simulink model "ControllerModelStateflow"  (R2022b)
settings: Solver=VariableStepAuto  StartTime=0.0  StopTime=inf  RelTol=1e-3
libraries: slpidlib x1
settings Model: Creator=steph  LastModifiedBy=steph
settings OptimizationCC: BlockReduction=off  DefaultParameterBehavior=Inlined  BufferReuse=off

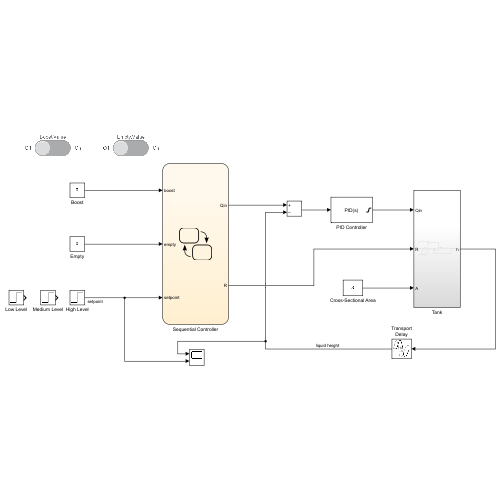
[thumbnail: Simulink's stored preview of the top-level diagram]
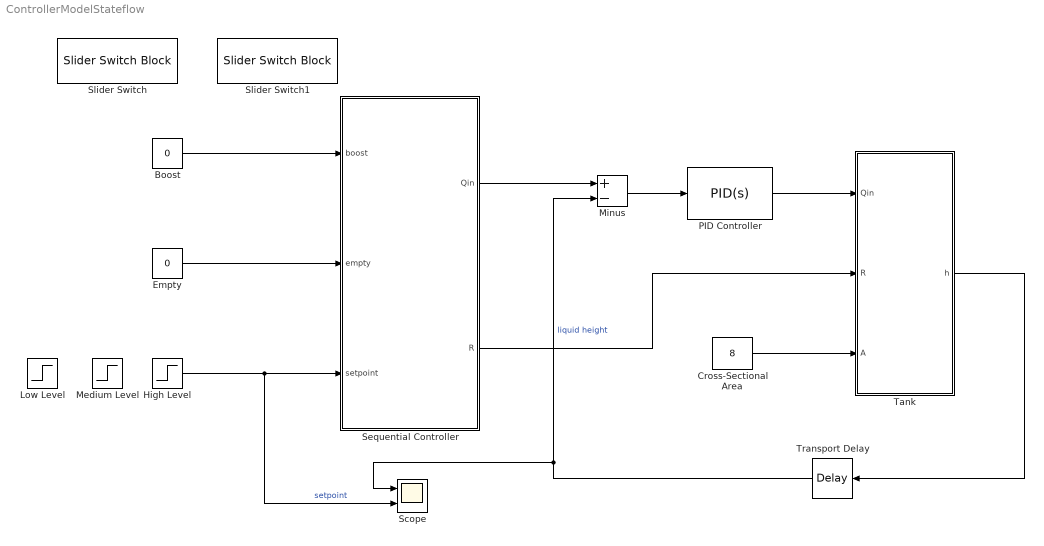
== system ControllerModelStateflow ==
  Boost : Constant  Value=0  OutMin=0  OutMax=1
  Cross-Sectional Area : Constant  Value=8  OutMin=0  OutMax=200
  Empty : Constant  Value=0  OutMin=0  OutMax=1
  High Level : Step  Time=4  After=16  SampleTime=0
  Low Level : Step  Time=0.25  After=2  SampleTime=0
  Medium Level : Step  Time=2  After=8  SampleTime=0
  Minus : Sum  Inputs=+-
  PID Controller : slpidlib/PID Controller  Controller=PID  Form=Parallel  TimeDomain=Continuous-time  UseExternalTs=off  SampleTime=-1  IntegratorMethod=Forward Euler  FilterMethod=Forward Euler  ControllerParametersSource=internal  P=0.6*8.25  I=2*(1/6.5)  UseKiTs=off  D=0.125/(1/2.3)  N=100  UseFilter=on  TunerSelectOption=Transfer Function Based (PID Tuner App)  InitialConditionSource=internal  InitialConditionForIntegrator=0  InitialConditionForFilter=0  DifferentiatorICPrevScaledInput=0  ExternalReset=none  TrackingMode=off  Kt=1  LimitOutput=on  SatLimitsSource=internal  UpperSaturationLimit=50  LowerSaturationLimit=0  LinearizeAsGain=on  AntiWindupMode=none  Kb=1  LimitIntegrator=off  UpperIntegratorSaturationLimit=inf  LowerIntegratorSaturationLimit=-inf  POutMin=[]  POutMax=[]  IOutMin=[]  IOutMax=[]  DOutMin=[]  DOutMax=[]  NOutMin=[]  NOutMax=[]  SumOutMin=[]  SumOutMax=[]  SaturationOutMin=[]  SaturationOutMax=[]  PParamMin=[]  PParamMax=[]  IParamMin=[]  IParamMax=[]  DParamMin=[]  DParamMax=[]  NParamMin=[]  NParamMax=[]  KbParamMin=[]  KbParamMax=[]  KtParamMin=[]  KtParamMax=[]  KbOutMin=[]  KbOutMax=[]  KtOutMin=[]  KtOutMax=[]  IntegratorOutMin=[]  IntegratorOutMax=[]  FilterOutMin=[]  FilterOutMax=[]  SumI1OutMin=[]  SumI1OutMax=[]  SumI2OutMin=[]  SumI2OutMax=[]  SumI3OutMin=[]  SumI3OutMax=[]  SumI4OutMin=[]  SumI4OutMax=[]  SumDOutMin=[]  SumDOutMax=[]  DifferentiatorOutMin=[]  DifferentiatorOutMax=[]  FilterDiffOutCoefMin=[]  FilterDiffOutCoefMax=[]  ReciprocalOutMin=[]  ReciprocalOutMax=[]  SumDenOutMin=[]  SumDenOutMax=[]  SumNumOutMin=[]  SumNumOutMax=[]  DivideOutMin=[]  DivideOutMax=[]  UdiffTsProdOutMin=[]  UdiffTsProdOutMax=[]  NTsProdOutMin=[]  NTsProdOutMax=[]  UintegralTsProdOutMin=[]  UintegralTsProdOutMax=[]  UngainTsProdOutMin=[]  UngainTsProdOutMax=[]  ClampingZeroOutDataTypeStr=Inherit: Inherit via back propagation  ClampingZeroOutMin=[]  ClampingZeroOutMax=[]  FilterDenConstantOutDataTypeStr=Inherit: Inherit via back propagation  FilterDenConstantOutMin=[]  FilterDenConstantOutMax=[]  PCopyOutDataTypeStr=Inherit: Inherit via back propagation  PCopyOutMin=[]  PCopyOutMax=[]  NCopyOutDataTypeStr=Inherit: Inherit via back propagation  NCopyOutMin=[]  NCopyOutMax=[]  IntegratorContinuousStateAttributes=''  IntegratorStateMustResolveToSignalObject=off  IntegratorRTWStateStorageClass=Auto  FilterContinuousStateAttributes=''  FilterStateMustResolveToSignalObject=off  FilterRTWStateStorageClass=Auto  ParallelPVariant=InternalParameters  IdealPVariant=Disabled  IVariant=InternalParameters  DVariant=InternalParameters  IntegratorVariant=Continuous  SatVariant=Enabled  AWVariant=Passthrough  PCopyVariant=Disabled  TRVariant=Disabled  FdbkBlocksVariant=Forward  IdealPFdbkVariant=Disabled  SatFdbkVariant=Disabled  DerivativeFilterVariant=ContFilter  NVariant=InternalParameters  NCopyVariant=Disabled  FilterICVariant=InternalICsFilter  IntegratorICVariant=InternalICs  ExternalResetVariant=Disabled  TRSumVariant=Passthrough  SumFdbkVariant=Disabled  SumVariant=Sum_PID  TsampFilterVariant=InternalTs  TsampNgainVariant=Passthrough  TsampIntegralVariant=Passthrough  ExternalSaturationOutDataTypeStr=Inherit: Same as second input
  Scope : Scope  NumInputPorts=2
  Sequential Controller : Stateflow chart  TreatAsAtomicUnit=on
  Slider Switch : SliderSwitchBlock
      settings: Values={{'Off', 'On'}, [0 1]}
  Slider Switch1 : SliderSwitchBlock
      settings: Values={{'Off', 'On'}, [0 1]}
  Tank : Subsystem
  Transport Delay : TransportDelay  DelayTime=0.05
  wires:
  Sequential Controller/2(R) -> Tank/2(R)
  Cross-Sectional Area/1 -> Tank/3(A)
  Tank/1(h) -> Transport Delay/1
  Transport Delay/1 -> Minus/2, Scope/1  "liquid height"
  Minus/1 -> PID Controller/1
  PID Controller/1 -> Tank/1(Qin)
  Sequential Controller/1(Qin) -> Minus/1
  Boost/1 -> Sequential Controller/1(boost)
  Empty/1 -> Sequential Controller/2(empty)
  High Level/1 -> Scope/2, Sequential Controller/3(setpoint)  "setpoint"

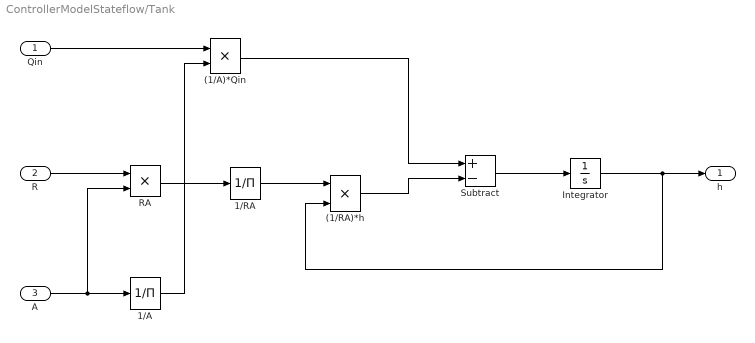
== system ControllerModelStateflow/Tank ==
  Qin : Inport
  R : Inport  Port=2
  A : Inport  Port=3
  (1/A)*Qin : Product
  (1/RA)*h : Product
  1/A : Product  Inputs=/
  1/RA : Product  Inputs=/
  Integrator : Integrator
  RA : Product
  Subtract : Sum  Inputs=+-
  h : Outport
  wires:
  A/1 -> RA/2, 1/A/1
  R/1 -> RA/1
  RA/1 -> 1/RA/1
  1/A/1 -> (1/A)*Qin/2
  1/RA/1 -> (1/RA)*h/1
  (1/A)*Qin/1 -> Subtract/1
  (1/RA)*h/1 -> Subtract/2
  Integrator/1 -> (1/RA)*h/2, h/1
  Qin/1 -> (1/A)*Qin/1
  Subtract/1 -> Integrator/1

== stateflow chart ControllerModelStateflow/Sequential Controller ==
  state Application
    state Init
      entry:
      Qin = setpoint;
      R=1;
    state Boost
      entry:
      Qin = setpoint*1.1;
      R=1;
    state Empty
      entry:
      R=0.001;
      Qin = 0;
    Empty -> Init [order 1] : [empty == 0 && after(5,sec)]
    Init -> Boost [order 1] : [boost == 1]
    Boost -> Init : [boost == 0 || after(10,sec)]
    Init -> Empty [order 2] : [empty == 1]
    Empty -> Boost [order 2] : [boost == 1]
  (default) -> Init
  data: boost input; empty input; Qin output; setpoint input; R output
